simulink model "week2_4"  (R2020b)
settings: Solver=ode45  StartTime=0.0  StopTime=10.0  RelTol=1e-3
undefined symbols (not defined in the file or in its folder): b, J, Ke, Kt, L, R
settings Model: Creator=sansh  LastModifiedBy=Lenovo
settings DataIOCC: ReturnWorkspaceOutputs=off
settings DebuggingCC: ArithmeticOperatorsInVariantConditions=warning
settings SFSimCC: SimUseLocalCustomCode=off  CustomCodeUndefinedFunction=UseInterfaceOnly
settings RTWCC: RTWUseLocalCustomCode=off
settings CodeAppCC: StateflowObjectComments=on

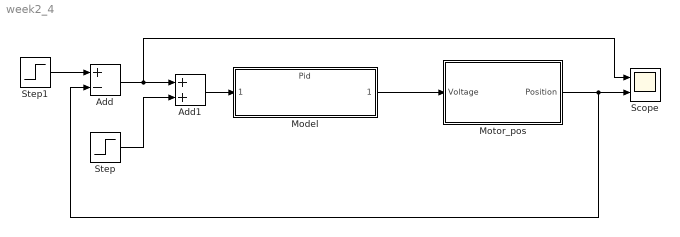
== system week2_4 ==
  Add : Sum  Inputs=+-
  Add1 : Sum
  Model : ModelReference  ModelNameDialog=Pid.slx  SimulationMode=Normal  ModelReferenceVersion=1.1
  Motor_pos : Subsystem
  Scope : Scope  NumInputPorts=2
  Step : Step  Time=0.01  After=0.1  SampleTime=0
  Step1 : Step  Time=0.01  SampleTime=0
  wires:
  Step1/1 -> Add/1
  Motor_pos/1(Position) -> Add/2, Scope/2
  Add/1 -> Scope/1, Add1/1
  Model/1 -> Motor_pos/1(Voltage)
  Step/1 -> Add1/2
  Add1/1 -> Model/1

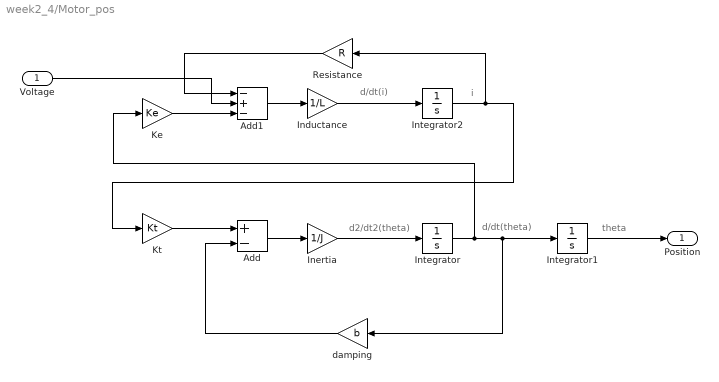
== system week2_4/Motor_pos ==
  note: i
  note: d/dt(i)
  note: d2/dt2(theta)
  note: d/dt(theta)
  note: theta
  Voltage : Inport
  Add : Sum  Inputs=+-
  Add1 : Sum  Inputs=-+-
  Inductance : Gain  Gain=1/L
  Inertia : Gain  Gain=1/J
  Integrator : Integrator
  Integrator1 : Integrator
  Integrator2 : Integrator
  Ke : Gain  Gain=Ke
  Kt : Gain  Gain=Kt
  Resistance : Gain  Gain=R
  damping : Gain  Gain=b
  Position : Outport
  wires:
  Inertia/1 -> Integrator/1
  Inductance/1 -> Integrator2/1
  Integrator2/1 -> Resistance/1, Kt/1
  Integrator/1 -> Ke/1, damping/1, Integrator1/1
  Integrator1/1 -> Position/1
  Voltage/1 -> Add1/2
  Add/1 -> Inertia/1
  damping/1 -> Add/2
  Kt/1 -> Add/1
  Resistance/1 -> Add1/1
  Ke/1 -> Add1/3
  Add1/1 -> Inductance/1
